simulink model "untitled"  (R2020a)
settings: Solver=VariableStepAuto  StartTime=0.0  StopTime=10.0  RelTol=1e-3
libraries: simulink x1, dsparch4 x1
settings Model: Creator=93548  LastModifiedBy=93548

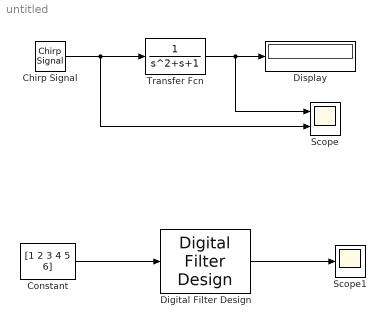
== system untitled ==
  Chirp Signal : simulink/Sources/Chirp Signal  f1=0.1  T=100  f2=1
  Constant : Constant  Value=[1 2 3 4 5 6]
  Digital Filter Design : dsparch4/Digital Filter Design  mwdsp_browser_bugfix_var=off
  Display : Display
  Scope : Scope  NumInputPorts=2
  Scope1 : Scope
  Transfer Fcn : TransferFcn  Denominator=[1 1 1]  ContinuousStateAttributes='pos'
  wires:
  Chirp Signal/1 -> Scope/2, Transfer Fcn/1
  Transfer Fcn/1 -> Scope/1, Display/1
  Constant/1 -> Digital Filter Design/1
  Digital Filter Design/1 -> Scope1/1
